simulink model "EposDemo2"  (R2020b)
settings: Solver=VariableStepAuto  StartTime=0.0  StopTime=10.0  RelTol=1e-3
InitFcn:
  | DemoEpos2_Init
libraries: sldrtlib x1
settings Model: Creator=Wacom hrg  LastModifiedBy=Wacom hrg

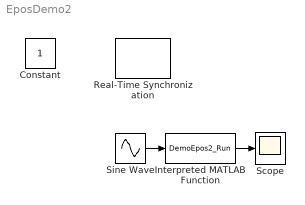
== system EposDemo2 ==
  Interpreted MATLAB Function : MATLABFcn  MATLABFcn=DemoEpos2_Run
  Real-Time Synchronization : sldrtlib/Real-Time Synchronization  SampleTime=0.1  MaxMissedTicks=10  ShowMissedTicks=off  YieldWhenWaiting=off
  Scope : Scope
  Sine Wave : Sin  SampleTime=0
  Constant : Constant  IOType=siggen
  wires:
  Sine Wave/1 -> Interpreted MATLAB Function/1
  Interpreted MATLAB Function/1 -> Scope/1
